simulink model "mount_2_rust"  (R2022b)
settings: Solver=FixedStepDiscrete  StartTime=0.0  StopTime=5  FixedStep=deltaT  RelTol=1e-3
InitFcn:
  | %
  | % Initialization callback function
  | %
  | 
  | try
  |    % fprintf('\n Simulink control model!\n');
  | 
  |    % Get Simulink model directory
  |    [filepath,name,ext] = fileparts(which(bdroot));
  | 
  |    if ~strcmp(filepath,pwd)
  |       fprintf('\n Changing current directory to \n %s \n',filepath);
  |       cd(filepath);
  |    end
  | 
  | catch
  |    warning('Running the InitFcn from puSimulate script');
  | end
values from neighbouring files (symbols this model uses):
  drv_delay = ceil(mount.delay/FEM_Ts)    [load_mount_data.m]
  FEM_Ts = deltaT    (= 0.000125)    [load_mount_data.m]
  Hdrive_d = c2d(o.Hdrive(1,1), FEM_Ts, 'tustin')    [load_mount_data.m]
  mnt_TF_Ts = FEM_Ts    (= 0.000125)    [load_mount_data.m]
  o = fun_confBase(oTest)    [load_mount_data.m]
undefined symbols (not defined in the file or in its folder): a, az, az_ff_en, b, c, DiscIntNeverNeededParam, el, gir, magnitude, mount
libraries: simulink x2, simulink_extras x2
(part 2 of 2)

== system mount_2_rust/Mount_Drv_PDR2021/ODC CT LUGRE Fr model/Friction ==
  Vel : Inport
  Enable : EnablePort
  Constant : Constant  Value=az.oFr.iIsActive
  Constant1 : Constant  Value=el.oFr.iIsActive
  Constant2 : Constant  Value=gir.oFr.iIsActive
  Demux1 : Demux  Outputs=3
  Friction Alt : Subsystem  mask{sigma0=el.oFr.sigm0, sigma1=el.oFr.sigm1, Tc=el.oFr.Tc, sigmav=el.oFr.sigmv, Ts=el.oFr.Ts, vs=el.oFr.vs, iIsSig01Active=el.oFr.iIsSig01Active}
      mask prompts: iIsSig01Active "0=inactive, 1=active"
  Friction Az : Subsystem  mask{sigma0=az.oFr.sigm0, sigma1=az.oFr.sigm1, Tc=az.oFr.Tc, sigmav=az.oFr.sigmv, Ts=az.oFr.Ts, vs=az.oFr.vs, iIsSig01Active=az.oFr.iIsSig01Active}
      mask prompts: iIsSig01Active "0=inactive, 1=active"
  Friction Gir : Subsystem  mask{sigma0=gir.oFr.sigm0, sigma1=gir.oFr.sigm1, Tc=gir.oFr.Tc, sigmav=gir.oFr.sigmv, Ts=gir.oFr.Ts, vs=gir.oFr.vs, iIsSig01Active=gir.oFr.iIsSig01Active}
      mask prompts: iIsSig01Active "0=inactive, 1=active"
  Mux2 : Mux  Inputs=3
  FrictionTo : Outport
  wires:
  Friction Gir/1(Tfr) -> Mux2/3
  Demux1/3 -> Friction Gir/1(v)
  Constant2/1 -> Friction Gir/Enable
  Constant/1 -> Friction Az/Enable
  Constant1/1 -> Friction Alt/Enable
  Mux2/1 -> FrictionTo/1
  Friction Az/1(Tfr) -> Mux2/1
  Demux1/1 -> Friction Az/1(v)
  Vel/1 -> Demux1/1
  Demux1/2 -> Friction Alt/1(v)
  Friction Alt/1(Tfr) -> Mux2/2

== system mount_2_rust/Mount_Drv_PDR2021/Parasitic torques model /AZ_Parasitic_Torque ==
  Drive_Pos : Inport
  Drive_Torque : Inport  Port=2
  Cogging : Lookup_n-D  NumberOfTableDimensions=1  LookupTableObject=F_ripple  BreakpointsForDimension1=ParasiticModelStruc.Pos  Table=ParasiticModelStruc.oCog.Amp  InternalRulePriority=Speed  RndMeth=Simplest
  Constant : Constant  Value=0.1869
  Divide : Product  Inputs=**
  EMF Distortion : Lookup_n-D  NumberOfTableDimensions=1  LookupTableObject=F_ripple  BreakpointsForDimension1=ParasiticModelStruc.Pos  Table=ParasiticModelStruc.oEmf.Amp  InternalRulePriority=Speed  RndMeth=Simplest
  Gain : Gain  Gain=1/ParasiticModelStruc.R
  Gain1 : Gain  Gain=1/250
  Gain2 : Gain  Gain=1/ParasiticModelStruc.N_Segm
  Mod : Math  Operator=rem  SignedPower=on
  Mod1 : Math  Operator=rem  SignedPower=on
  Radius : Gain  Gain=ParasiticModelStruc.R
  Sum1 : Sum
  Sum2 : Sum
  Parasitic_Torque : Outport  VectorParamsAs1DForOutWhenUnconnected=off
  wires:
  Sum1/1 -> Parasitic_Torque/1
  Drive_Pos/1 -> Radius/1  "Drive Position"
  Constant/1 -> Mod1/2, Sum2/2, Mod/2
  Gain2/1 -> Divide/1  "I_rms pro Segment"
  Mod/1 -> Sum2/1
  Sum2/1 -> Mod1/1
  EMF Distortion/1 -> Divide/2
  Gain/1 -> Gain1/1  "Force"
  Drive_Torque/1 -> Gain/1
  Radius/1 -> Mod/1  "driven  distance"
  Cogging/1 -> Sum1/2
  Mod1/1 -> Cogging/1, EMF Distortion/1
  Gain1/1 -> Gain2/1  "I_rms"
  Divide/1 -> Sum1/1

== system mount_2_rust/Mount_Drv_PDR2021/Parasitic torques model /EL_Parasitic_Torque ==
  Drive_Pos : Inport
  Drive_Torque : Inport  Port=2
  Cogging : Lookup_n-D  NumberOfTableDimensions=1  LookupTableObject=F_ripple  BreakpointsForDimension1=ParasiticModelStruc.Pos  Table=ParasiticModelStruc.oCog.Amp  InternalRulePriority=Speed  RndMeth=Simplest
  Constant : Constant  Value=0.1869
  Divide : Product  Inputs=**
  EMF Distortion : Lookup_n-D  NumberOfTableDimensions=1  LookupTableObject=F_ripple  BreakpointsForDimension1=ParasiticModelStruc.Pos  Table=ParasiticModelStruc.oEmf.Amp  InternalRulePriority=Speed  RndMeth=Simplest
  Gain : Gain  Gain=1/ParasiticModelStruc.R
  Gain1 : Gain  Gain=1/250
  Gain2 : Gain  Gain=1/ParasiticModelStruc.N_Segm
  Mod : Math  Operator=rem  SignedPower=on
  Mod1 : Math  Operator=rem  SignedPower=on
  Radius : Gain  Gain=ParasiticModelStruc.R
  Sum1 : Sum
  Sum2 : Sum
  Parasitic_Torque : Outport  VectorParamsAs1DForOutWhenUnconnected=off
  wires:
  Constant/1 -> Mod1/2, Sum2/2, Mod/2
  Divide/1 -> Sum1/1
  Mod1/1 -> Cogging/1, EMF Distortion/1
  Sum2/1 -> Mod1/1
  Radius/1 -> Mod/1  "driven  distance"
  Cogging/1 -> Sum1/2
  Mod/1 -> Sum2/1
  Gain/1 -> Gain1/1  "Force"
  Gain2/1 -> Divide/1  "I_rms pro Segment"
  Gain1/1 -> Gain2/1  "I_rms"
  Drive_Pos/1 -> Radius/1  "Drive Position"
  EMF Distortion/1 -> Divide/2
  Drive_Torque/1 -> Gain/1
  Sum1/1 -> Parasitic_Torque/1

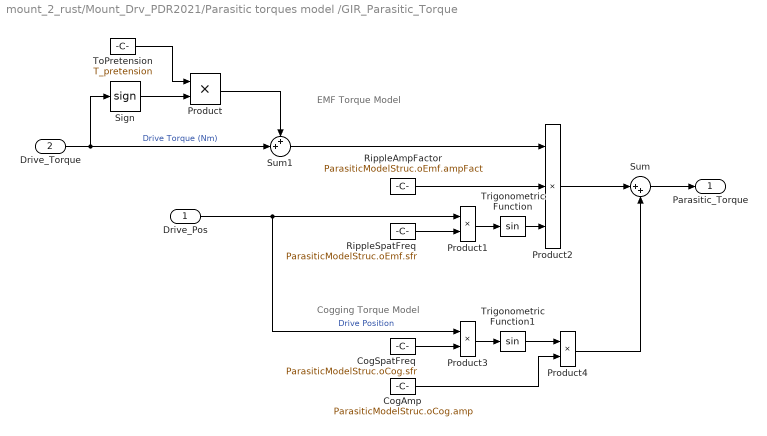
== system mount_2_rust/Mount_Drv_PDR2021/Parasitic torques model /GIR_Parasitic_Torque ==
  note: Cogging Torque Model
  note: EMF Torque Model
  Drive_Pos : Inport
  Drive_Torque : Inport  Port=2
  CogAmp : Constant  Value=ParasiticModelStruc.oCog.amp
  CogSpatFreq : Constant  Value=ParasiticModelStruc.oCog.sfr
  Product : Product
  Product1 : Product  RndMeth=Zero
  Product2 : Product  Inputs=3  RndMeth=Zero
  Product3 : Product  RndMeth=Zero
  Product4 : Product  RndMeth=Zero
  RippleAmpFactor : Constant  Value=ParasiticModelStruc.oEmf.ampFact
  RippleSpatFreq : Constant  Value=ParasiticModelStruc.oEmf.sfr
  Sign : Signum
  Sum : Sum  Inputs=|++
  Sum1 : Sum  Inputs=++|
  ToPretension : Constant  Value=T_pretension
  Trigonometric Function : Trigonometry
  Trigonometric Function1 : Trigonometry
  Parasitic_Torque : Outport  VectorParamsAs1DForOutWhenUnconnected=off
  wires:
  Product/1 -> Sum1/1
  ToPretension/1 -> Product/1
  Sign/1 -> Product/2
  Drive_Torque/1 -> Sum1/2, Sign/1  "Drive Torque (Nm)"
  Sum1/1 -> Product2/1
  Trigonometric Function/1 -> Product2/3
  Sum/1 -> Parasitic_Torque/1
  Product2/1 -> Sum/1
  Product4/1 -> Sum/2
  CogAmp/1 -> Product4/2
  Drive_Pos/1 -> Product1/1, Product3/1  "Drive Position"
  CogSpatFreq/1 -> Product3/2
  Trigonometric Function1/1 -> Product4/1
  Product3/1 -> Trigonometric Function1/1
  RippleSpatFreq/1 -> Product1/2
  Product1/1 -> Trigonometric Function/1
  RippleAmpFactor/1 -> Product2/2

== system mount_2_rust/Mount_Drv_PDR2021/Parasitic torques model /Subsystem ==
  Az Pos : Inport
  Az To : Inport  Port=2
  El Pos : Inport  Port=3
  El To : Inport  Port=4
  Gir Pos : Inport  Port=5
  Gir To : Inport  Port=6
  Constant2 : Constant
  Demux1 : Demux  Outputs=3
  Mux1 : Mux  Inputs=3
  Mux7 : Mux  Inputs=3
  Parasitic Torques : Subsystem
  Out1 : Outport  VectorParamsAs1DForOutWhenUnconnected=off
  Out2 : Outport  Port=2  VectorParamsAs1DForOutWhenUnconnected=off
  Out3 : Outport  Port=3  VectorParamsAs1DForOutWhenUnconnected=off
  wires:
  Gir To/1 -> Mux1/3
  El To/1 -> Mux1/2
  Az To/1 -> Mux1/1
  Parasitic Torques/1(ParasiticTo) -> Demux1/1
  El Pos/1 -> Mux7/2
  Constant2/1 -> Parasitic Torques/Enable
  Mux1/1 -> Parasitic Torques/1(MotTo)
  Mux7/1 -> Parasitic Torques/2(MotPos)
  Az Pos/1 -> Mux7/1
  Demux1/3 -> Out3/1
  Gir Pos/1 -> Mux7/3
  Demux1/2 -> Out2/1
  Demux1/1 -> Out1/1

== system mount_2_rust/Mount_Drv_PDR2021_Frless/Parasitic torques model /AZ_Parasitic_Torque ==
  Drive_Pos : Inport
  Drive_Torque : Inport  Port=2
  Cogging : Lookup_n-D  NumberOfTableDimensions=1  LookupTableObject=F_ripple  BreakpointsForDimension1=ParasiticModelStruc.Pos  Table=ParasiticModelStruc.oCog.Amp  InternalRulePriority=Speed  RndMeth=Simplest
  Constant : Constant  Value=0.1869
  Divide : Product  Inputs=**
  EMF Distortion : Lookup_n-D  NumberOfTableDimensions=1  LookupTableObject=F_ripple  BreakpointsForDimension1=ParasiticModelStruc.Pos  Table=ParasiticModelStruc.oEmf.Amp  InternalRulePriority=Speed  RndMeth=Simplest
  Gain : Gain  Gain=1/ParasiticModelStruc.R
  Gain1 : Gain  Gain=1/250
  Gain2 : Gain  Gain=1/ParasiticModelStruc.N_Segm
  Mod : Math  Operator=rem  SignedPower=on
  Mod1 : Math  Operator=rem  SignedPower=on
  Radius : Gain  Gain=ParasiticModelStruc.R
  Sum1 : Sum
  Sum2 : Sum
  Parasitic_Torque : Outport  VectorParamsAs1DForOutWhenUnconnected=off
  wires:
  Sum1/1 -> Parasitic_Torque/1
  Drive_Pos/1 -> Radius/1  "Drive Position"
  Constant/1 -> Mod1/2, Sum2/2, Mod/2
  Gain2/1 -> Divide/1  "I_rms pro Segment"
  Mod/1 -> Sum2/1
  Sum2/1 -> Mod1/1
  EMF Distortion/1 -> Divide/2
  Gain/1 -> Gain1/1  "Force"
  Drive_Torque/1 -> Gain/1
  Radius/1 -> Mod/1  "driven  distance"
  Cogging/1 -> Sum1/2
  Mod1/1 -> Cogging/1, EMF Distortion/1
  Gain1/1 -> Gain2/1  "I_rms"
  Divide/1 -> Sum1/1

== system mount_2_rust/Mount_Drv_PDR2021_Frless/Parasitic torques model /EL_Parasitic_Torque ==
  Drive_Pos : Inport
  Drive_Torque : Inport  Port=2
  Cogging : Lookup_n-D  NumberOfTableDimensions=1  LookupTableObject=F_ripple  BreakpointsForDimension1=ParasiticModelStruc.Pos  Table=ParasiticModelStruc.oCog.Amp  InternalRulePriority=Speed  RndMeth=Simplest
  Constant : Constant  Value=0.1869
  Divide : Product  Inputs=**
  EMF Distortion : Lookup_n-D  NumberOfTableDimensions=1  LookupTableObject=F_ripple  BreakpointsForDimension1=ParasiticModelStruc.Pos  Table=ParasiticModelStruc.oEmf.Amp  InternalRulePriority=Speed  RndMeth=Simplest
  Gain : Gain  Gain=1/ParasiticModelStruc.R
  Gain1 : Gain  Gain=1/250
  Gain2 : Gain  Gain=1/ParasiticModelStruc.N_Segm
  Mod : Math  Operator=rem  SignedPower=on
  Mod1 : Math  Operator=rem  SignedPower=on
  Radius : Gain  Gain=ParasiticModelStruc.R
  Sum1 : Sum
  Sum2 : Sum
  Parasitic_Torque : Outport  VectorParamsAs1DForOutWhenUnconnected=off
  wires:
  Constant/1 -> Mod1/2, Sum2/2, Mod/2
  Divide/1 -> Sum1/1
  Mod1/1 -> Cogging/1, EMF Distortion/1
  Sum2/1 -> Mod1/1
  Radius/1 -> Mod/1  "driven  distance"
  Cogging/1 -> Sum1/2
  Mod/1 -> Sum2/1
  Gain/1 -> Gain1/1  "Force"
  Gain2/1 -> Divide/1  "I_rms pro Segment"
  Gain1/1 -> Gain2/1  "I_rms"
  Drive_Pos/1 -> Radius/1  "Drive Position"
  EMF Distortion/1 -> Divide/2
  Drive_Torque/1 -> Gain/1
  Sum1/1 -> Parasitic_Torque/1

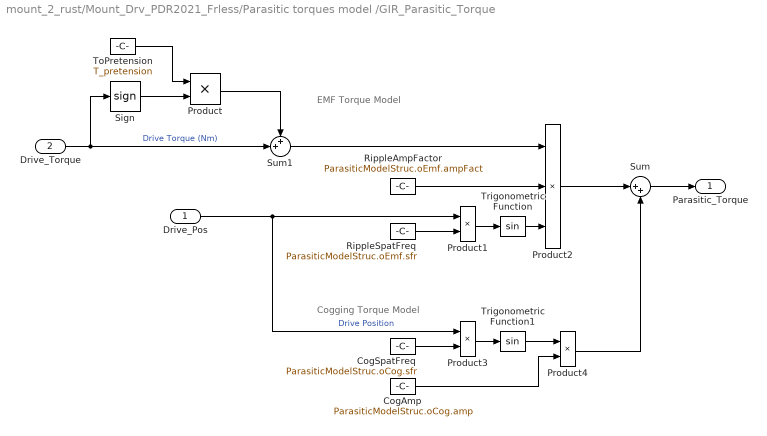
== system mount_2_rust/Mount_Drv_PDR2021_Frless/Parasitic torques model /GIR_Parasitic_Torque ==
  note: Cogging Torque Model
  note: EMF Torque Model
  Drive_Pos : Inport
  Drive_Torque : Inport  Port=2
  CogAmp : Constant  Value=ParasiticModelStruc.oCog.amp
  CogSpatFreq : Constant  Value=ParasiticModelStruc.oCog.sfr
  Product : Product
  Product1 : Product  RndMeth=Zero
  Product2 : Product  Inputs=3  RndMeth=Zero
  Product3 : Product  RndMeth=Zero
  Product4 : Product  RndMeth=Zero
  RippleAmpFactor : Constant  Value=ParasiticModelStruc.oEmf.ampFact
  RippleSpatFreq : Constant  Value=ParasiticModelStruc.oEmf.sfr
  Sign : Signum
  Sum : Sum  Inputs=|++
  Sum1 : Sum  Inputs=++|
  ToPretension : Constant  Value=T_pretension
  Trigonometric Function : Trigonometry
  Trigonometric Function1 : Trigonometry
  Parasitic_Torque : Outport  VectorParamsAs1DForOutWhenUnconnected=off
  wires:
  Product/1 -> Sum1/1
  ToPretension/1 -> Product/1
  Sign/1 -> Product/2
  Drive_Torque/1 -> Sum1/2, Sign/1  "Drive Torque (Nm)"
  Sum1/1 -> Product2/1
  Trigonometric Function/1 -> Product2/3
  Sum/1 -> Parasitic_Torque/1
  Product2/1 -> Sum/1
  Product4/1 -> Sum/2
  CogAmp/1 -> Product4/2
  Drive_Pos/1 -> Product1/1, Product3/1  "Drive Position"
  CogSpatFreq/1 -> Product3/2
  Trigonometric Function1/1 -> Product4/1
  Product3/1 -> Trigonometric Function1/1
  RippleSpatFreq/1 -> Product1/2
  Product1/1 -> Trigonometric Function/1
  RippleAmpFactor/1 -> Product2/2

== system mount_2_rust/Mount_Drv_PDR2021_Frless/Parasitic torques model /Subsystem ==
  Az Pos : Inport
  Az To : Inport  Port=2
  El Pos : Inport  Port=3
  El To : Inport  Port=4
  Gir Pos : Inport  Port=5
  Gir To : Inport  Port=6
  Constant2 : Constant
  Demux1 : Demux  Outputs=3
  Mux1 : Mux  Inputs=3
  Mux7 : Mux  Inputs=3
  Parasitic Torques : Subsystem
  Out1 : Outport  VectorParamsAs1DForOutWhenUnconnected=off
  Out2 : Outport  Port=2  VectorParamsAs1DForOutWhenUnconnected=off
  Out3 : Outport  Port=3  VectorParamsAs1DForOutWhenUnconnected=off
  wires:
  Gir To/1 -> Mux1/3
  El To/1 -> Mux1/2
  Az To/1 -> Mux1/1
  Parasitic Torques/1(ParasiticTo) -> Demux1/1
  El Pos/1 -> Mux7/2
  Constant2/1 -> Parasitic Torques/Enable
  Mux1/1 -> Parasitic Torques/1(MotTo)
  Mux7/1 -> Parasitic Torques/2(MotPos)
  Az Pos/1 -> Mux7/1
  Demux1/3 -> Out3/1
  Gir Pos/1 -> Mux7/3
  Demux1/2 -> Out2/1
  Demux1/1 -> Out1/1

== system mount_2_rust/Mount_Drv_FDR2023/DRV Friction/AZ DT Lugre Fr mode/g(v) ==
  v : Inport
  Enable : EnablePort
  Constant : Constant  Value=0
  Sum : Sum  Inputs=|++
  gc : Constant  Value=Tc/sigma0
  gs : Subsystem
  g : Outport
  wires:
  Constant/1 -> gs/Enable
  gc/1 -> Sum/2
  gs/1(gs(v)) -> Sum/1
  v/1 -> gs/1(v)
  Sum/1 -> g/1

== system mount_2_rust/Mount_Drv_FDR2023/DRV Friction/AZ DT Lugre Fr mode/v2z ==
  v : Inport
  g(v) : Inport  Port=2
  z : Inport  Port=3
  Enable : EnablePort
  Abs : Abs  SaturateOnIntegerOverflow=off
  Divide : Product  Inputs=*/*
  Sum : Sum  Inputs=|+-
  dz : Outport
  wires:
  z/1 -> Divide/3
  g(v)/1 -> Divide/2
  Sum/1 -> dz/1
  v/1 -> Abs/1, Sum/1
  Divide/1 -> Sum/2
  Abs/1 -> Divide/1

== system mount_2_rust/Mount_Drv_FDR2023/DRV Friction/EL DT Lugre Fr model/g(v) ==
  v : Inport
  Enable : EnablePort
  Constant : Constant  Value=0
  Sum : Sum  Inputs=|++
  gc : Constant  Value=Tc/sigma0
  gs : Subsystem
  g : Outport
  wires:
  Constant/1 -> gs/Enable
  gc/1 -> Sum/2
  gs/1(gs(v)) -> Sum/1
  v/1 -> gs/1(v)
  Sum/1 -> g/1

== system mount_2_rust/Mount_Drv_FDR2023/DRV Friction/EL DT Lugre Fr model/v2z ==
  v : Inport
  g(v) : Inport  Port=2
  z : Inport  Port=3
  Enable : EnablePort
  Abs : Abs  SaturateOnIntegerOverflow=off
  Divide : Product  Inputs=*/*
  Sum : Sum  Inputs=|+-
  dz : Outport
  wires:
  z/1 -> Divide/3
  g(v)/1 -> Divide/2
  Sum/1 -> dz/1
  v/1 -> Abs/1, Sum/1
  Divide/1 -> Sum/2
  Abs/1 -> Divide/1

== system mount_2_rust/Mount_Drv_FDR2023/DRV Friction/EL DT Lugre Fr model_/g(v) ==
  v : Inport
  Enable : EnablePort
  Constant : Constant  Value=0
  Sum : Sum  Inputs=|++
  gc : Constant  Value=frParStruct.Tc/frParStruct.sigm0
  gs : Subsystem
  g : Outport  VectorParamsAs1DForOutWhenUnconnected=off
  wires:
  Constant/1 -> gs/Enable
  gc/1 -> Sum/2
  gs/1(gs(v)) -> Sum/1
  v/1 -> gs/1(v)
  Sum/1 -> g/1

== system mount_2_rust/Mount_Drv_FDR2023/DRV Friction/EL DT Lugre Fr model_/v2z ==
  v : Inport
  g(v) : Inport  Port=2
  z : Inport  Port=3
  Enable : EnablePort
  Abs : Abs  SaturateOnIntegerOverflow=off
  Divide : Product  Inputs=*/*
  Sum : Sum  Inputs=|+-
  dz : Outport  VectorParamsAs1DForOutWhenUnconnected=off
  wires:
  z/1 -> Divide/3
  g(v)/1 -> Divide/2
  Sum/1 -> dz/1
  v/1 -> Abs/1, Sum/1
  Divide/1 -> Sum/2
  Abs/1 -> Divide/1

== system mount_2_rust/Mount_Drv_FDR2023/DRV Friction/GIR DT Lugre Fr model/g(v) ==
  v : Inport
  Constant : Constant  Value=0
  Sum : Sum  Inputs=|++
  gc : Constant  Value=Tc/sigma0
  gs : Subsystem
  g : Outport
  wires:
  Constant/1 -> gs/Enable
  gc/1 -> Sum/2
  gs/1(gs(v)) -> Sum/1
  v/1 -> gs/1(v)
  Sum/1 -> g/1

== system mount_2_rust/Mount_Drv_FDR2023/DRV Friction/GIR DT Lugre Fr model/v2z ==
  v : Inport
  g(v) : Inport  Port=2
  z : Inport  Port=3
  Abs : Abs  SaturateOnIntegerOverflow=off
  Divide : Product  Inputs=*/*
  Sum : Sum  Inputs=|+-
  dz : Outport
  wires:
  z/1 -> Divide/3
  g(v)/1 -> Divide/2
  Sum/1 -> dz/1
  v/1 -> Abs/1, Sum/1
  Divide/1 -> Sum/2
  Abs/1 -> Divide/1

== system mount_2_rust/Mount_Drv_FDR2023/DRV Friction/GIR DT Lugre Fr model_/g(v) ==
  v : Inport
  Constant : Constant  Value=0
  Sum : Sum  Inputs=|++
  gc : Constant  Value=frParStruct.Tc/frParStruct.sigm0
  gs : Subsystem
  g : Outport  VectorParamsAs1DForOutWhenUnconnected=off
  wires:
  Constant/1 -> gs/Enable
  gc/1 -> Sum/2
  gs/1(gs(v)) -> Sum/1
  v/1 -> gs/1(v)
  Sum/1 -> g/1

== system mount_2_rust/Mount_Drv_FDR2023/DRV Friction/GIR DT Lugre Fr model_/v2z ==
  note: $\text{Let}\\ |v| = v \sign(v) \\ \text{Sign function approximation:}\\ S_0(v) = \frac{2}{\pi}\atan(k_v v) \\ \text{Then, one approximates the original LuGre model equation}\\ \dot{z} = v - \frac{|v|}{g(v)}z \\ \text{with} \\ \dot{z} = vS_0^2(v) - \frac{vS_0(v)}{g(v)}z .$
  note: Original implementation
  v : Inport
  g(v) : Inport  Port=2
  z : Inport  Port=3
  2/pi : Gain  Gain=2/pi
  Abs1 : Abs  SaturateOnIntegerOverflow=off
  Divide : Product  Inputs=*/*
  Divide1 : Product  Inputs=*/*
  Divide2 : Product  Inputs=**
  Divide3 : Product  Inputs=**
  Math Function : Math  Operator=square  SignedPower=on
  Smoothed-Discontinuous Lugre Model Switch : ManualSwitch
  Sum : Sum  Inputs=|+-
  Sum1 : Sum  Inputs=|+-
  Trigonometric Function : Trigonometry  Operator=atan
  kv : Gain  Gain=1e6%1e-6
  dz : Outport  VectorParamsAs1DForOutWhenUnconnected=off
  wires:
  Smoothed-Discontinuous Lugre Model Switch/1 -> dz/1
  Sum/1 -> Smoothed-Discontinuous Lugre Model Switch/1  "Smoothed Lugre"
  Divide2/1 -> Sum/1
  Divide3/1 -> Divide/1  "S_2"
  Math Function/1 -> Divide2/2  "S_1"
  2/pi/1 -> Math Function/1, Divide3/1  "S_0"
  kv/1 -> Trigonometric Function/1
  Trigonometric Function/1 -> 2/pi/1
  v/1 -> Divide2/1, kv/1, Divide3/2, Sum1/1, Abs1/1
  z/1 -> Divide/3, Divide1/3
  Sum1/1 -> Smoothed-Discontinuous Lugre Model Switch/2  "Discontinuous"
  Abs1/1 -> Divide1/1
  g(v)/1 -> Divide/2, Divide1/2
  Divide1/1 -> Sum1/2
  Divide/1 -> Sum/2

== system mount_2_rust/Mount_Drv_FDR2023/Parasitic torque model/Parasitic AZ/For Each Subsystem ==
  In1 : Inport  Partition=on  PartitionDimension=1  PartitionWidth=1  PartitionOffset=0
  EMF Spatial Pattern (N/A) : Sin  TimeSource=Use external signal  Amplitude=oParasitic.oEmf.SpAmp_NPerA  Frequency=oParasitic.oEmf.SpFreq_mmInv*2*pi  Phase=oParasitic.oEmf.SpPhase_rad  SampleTime=0
  For Each : ForEach  DisableCoverage=on
  Sum of Elements2 : Sum  Inputs=+
  Out1 : Outport  ConcatenationDimension=1
  wires:
  Sum of Elements2/1 -> Out1/1
  In1/1 -> EMF Spatial Pattern (N/A)/1
  EMF Spatial Pattern (N/A)/1 -> Sum of Elements2/1

== system mount_2_rust/Mount_Drv_FDR2023/Parasitic torque model/Parasitic AZ/For Each Subsystem1 ==
  In1 : Inport  Partition=on  PartitionDimension=1  PartitionWidth=1  PartitionOffset=0
  Cogging Spatial Pattern (N) : Sin  TimeSource=Use external signal  Amplitude=oParasitic.oCog.SpAmp_N  Frequency=oParasitic.oCog.SpFreq_mmInv*2*pi  Phase=oParasitic.oCog.SpPhase_rad  SampleTime=0
  For Each : ForEach  DisableCoverage=on
  Sum of Elements2 : Sum  Inputs=+
  Out1 : Outport  ConcatenationDimension=1
  wires:
  Sum of Elements2/1 -> Out1/1
  In1/1 -> Cogging Spatial Pattern (N)/1
  Cogging Spatial Pattern (N)/1 -> Sum of Elements2/1

== system mount_2_rust/Mount_Drv_FDR2023/Parasitic torque model/Parasitic EL/For Each Subsystem ==
  In1 : Inport  Partition=on  PartitionDimension=1  PartitionWidth=1  PartitionOffset=0
  EMF Spatial Pattern (N/A) : Sin  TimeSource=Use external signal  Amplitude=oParasitic.oEmf.SpAmp_NPerA  Frequency=oParasitic.oEmf.SpFreq_mmInv*2*pi  Phase=oParasitic.oEmf.SpPhase_rad  SampleTime=0
  For Each : ForEach  DisableCoverage=on
  Sum of Elements2 : Sum  Inputs=+
  Out1 : Outport  ConcatenationDimension=1
  wires:
  Sum of Elements2/1 -> Out1/1
  In1/1 -> EMF Spatial Pattern (N/A)/1
  EMF Spatial Pattern (N/A)/1 -> Sum of Elements2/1

== system mount_2_rust/Mount_Drv_FDR2023/Parasitic torque model/Parasitic EL/For Each Subsystem1 ==
  In1 : Inport  Partition=on  PartitionDimension=1  PartitionWidth=1  PartitionOffset=0
  Cogging Spatial Pattern (N) : Sin  TimeSource=Use external signal  Amplitude=oParasitic.oCog.SpAmp_N  Frequency=oParasitic.oCog.SpFreq_mmInv*2*pi  Phase=oParasitic.oCog.SpPhase_rad  SampleTime=0
  For Each : ForEach  DisableCoverage=on
  Sum of Elements2 : Sum  Inputs=+
  Out1 : Outport  ConcatenationDimension=1
  wires:
  Sum of Elements2/1 -> Out1/1
  In1/1 -> Cogging Spatial Pattern (N)/1
  Cogging Spatial Pattern (N)/1 -> Sum of Elements2/1

== system mount_2_rust/Mount_Drv_FDR2023/Parasitic torque model/Parasitic GIR/For Each Subsystem ==
  In1 : Inport  Partition=on  PartitionDimension=1  PartitionWidth=1  PartitionOffset=0
  (N/A) : Sin  TimeSource=Use external signal  Amplitude=oParasitic.oEmf.SpAmp_NmPerA  Frequency=oParasitic.oEmf.SpFreq_degInv*2*pi  Phase=oParasitic.oEmf.SpPhase_rad  SampleTime=0
  For Each : ForEach  DisableCoverage=on
  Sum of Elements2 : Sum  Inputs=+
  Out1 : Outport  ConcatenationDimension=1
  wires:
  Sum of Elements2/1 -> Out1/1
  In1/1 -> (N/A)/1
  (N/A)/1 -> Sum of Elements2/1

== system mount_2_rust/Mount_Drv_FDR2023/Parasitic torque model/Parasitic GIR/For Each Subsystem1 ==
  In1 : Inport  Partition=on  PartitionDimension=1  PartitionWidth=1  PartitionOffset=0
  Cogging Spatial Pattern (N) : Sin  TimeSource=Use external signal  Amplitude=oParasitic.oCog.SpAmp_Nm  Frequency=oParasitic.oCog.SpFreq_degInv*2*pi  Phase=oParasitic.oCog.SpPhase_rad  SampleTime=0
  For Each : ForEach  DisableCoverage=on
  Sum of Elements2 : Sum  Inputs=+
  Out1 : Outport  ConcatenationDimension=1
  wires:
  Sum of Elements2/1 -> Out1/1
  In1/1 -> Cogging Spatial Pattern (N)/1
  Cogging Spatial Pattern (N)/1 -> Sum of Elements2/1

== system mount_2_rust/Mount_Drv_PDR2021/AZ DT Lugre Fr model/g(v)/gs ==
  v : Inport
  Enable : EnablePort
  Divide : Product  Inputs=**
  Gain : Gain  Gain=1/frParStruct.vs
  Math Function : Math  SignedPower=on
  Math Function1 : Math  Operator=magnitude^2  SignedPower=on
  Sum : Sum  Inputs=|++
  Unary Minus : UnaryMinus
  gc : Constant  Value=frParStruct.Tc/frParStruct.sigm0
  gs : Constant  Value=(frParStruct.Ts-frParStruct.Tc)/frParStruct.sigm0
  gs(v) : Outport  VectorParamsAs1DForOutWhenUnconnected=off
  wires:
  Sum/1 -> gs(v)/1
  Divide/1 -> Sum/1
  gc/1 -> Sum/2
  v/1 -> Gain/1
  Gain/1 -> Math Function1/1
  Unary Minus/1 -> Math Function/1
  Math Function1/1 -> Unary Minus/1
  gs/1 -> Divide/2
  Math Function/1 -> Divide/1

== system mount_2_rust/Mount_Drv_PDR2021/EL DT Lugre Fr model/g(v)/gs ==
  v : Inport
  Enable : EnablePort
  Divide : Product  Inputs=**
  Gain : Gain  Gain=1/frParStruct.vs
  Math Function : Math  SignedPower=on
  Math Function1 : Math  Operator=magnitude^2  SignedPower=on
  Unary Minus : UnaryMinus
  gs : Constant  Value=(frParStruct.Ts-frParStruct.Tc)/frParStruct.sigm0
  gs(v) : Outport  VectorParamsAs1DForOutWhenUnconnected=off
  wires:
  Divide/1 -> gs(v)/1
  v/1 -> Gain/1
  Gain/1 -> Math Function1/1
  Unary Minus/1 -> Math Function/1
  Math Function1/1 -> Unary Minus/1
  gs/1 -> Divide/2
  Math Function/1 -> Divide/1

== system mount_2_rust/Mount_Drv_PDR2021/GIR DT Lugre Fr model/g(v)/gs ==
  v : Inport
  Enable : EnablePort
  Divide : Product  Inputs=**
  Gain : Gain  Gain=1/frParStruct.vs
  Math Function : Math  SignedPower=on
  Math Function1 : Math  Operator=magnitude^2  SignedPower=on
  Unary Minus : UnaryMinus
  gs : Constant  Value=(frParStruct.Ts-frParStruct.Tc)/frParStruct.sigm0
  gs(v) : Outport  VectorParamsAs1DForOutWhenUnconnected=off
  wires:
  Divide/1 -> gs(v)/1
  v/1 -> Gain/1
  Gain/1 -> Math Function1/1
  Unary Minus/1 -> Math Function/1
  Math Function1/1 -> Unary Minus/1
  gs/1 -> Divide/2
  Math Function/1 -> Divide/1

== system mount_2_rust/Mount_Drv_PDR2021/ODC CT LUGRE Fr model/Friction/Friction Alt ==
  v : Inport
  Enable : EnablePort
  Constant : Constant  Value=iIsSig01Active
  Integrator2 : Integrator
  Sum : Sum  Inputs=+++
  g(v) : Subsystem
  sigma_0 : Gain  Gain=sigma0
  sigma_1 : Gain  Gain=sigma1
  sigma_v : Gain  Gain=sigmav
  v2z : Subsystem
  Tfr : Outport
  wires:
  Constant/1 -> g(v)/Enable, v2z/Enable
  v/1 -> sigma_v/1, v2z/1(v), g(v)/1(v)
  sigma_v/1 -> Sum/3
  sigma_1/1 -> Sum/1
  Sum/1 -> Tfr/1
  sigma_0/1 -> Sum/2
  g(v)/1(g) -> v2z/2(g(v))
  Integrator2/1 -> v2z/3(z), sigma_0/1
  v2z/1(dz) -> sigma_1/1, Integrator2/1

== system mount_2_rust/Mount_Drv_PDR2021/ODC CT LUGRE Fr model/Friction/Friction Az ==
  v : Inport
  Enable : EnablePort
  Constant : Constant  Value=iIsSig01Active
  Integrator2 : Integrator
  Sum : Sum  Inputs=+++
  g(v) : Subsystem
  sigma_0 : Gain  Gain=sigma0
  sigma_1 : Gain  Gain=sigma1
  sigma_v : Gain  Gain=sigmav
  v2z : Subsystem
  Tfr : Outport
  wires:
  Constant/1 -> v2z/Enable, g(v)/Enable
  v/1 -> sigma_v/1, v2z/1(v), g(v)/1(v)
  sigma_v/1 -> Sum/3
  sigma_1/1 -> Sum/1
  Sum/1 -> Tfr/1
  sigma_0/1 -> Sum/2
  g(v)/1(g) -> v2z/2(g(v))
  Integrator2/1 -> v2z/3(z), sigma_0/1
  v2z/1(dz) -> sigma_1/1, Integrator2/1

== system mount_2_rust/Mount_Drv_PDR2021/ODC CT LUGRE Fr model/Friction/Friction Gir ==
  v : Inport
  Enable : EnablePort
  Integrator2 : Integrator
  Sum : Sum  Inputs=+++
  g(v) : Subsystem
  iIsSig01Active : Gain  Gain=iIsSig01Active
  sigma_0 : Gain  Gain=sigma0
  sigma_1 : Gain  Gain=sigma1
  sigma_v : Gain  Gain=sigmav
  v2z : Subsystem
  Tfr : Outport
  wires:
  iIsSig01Active/1 -> v2z/1(v), g(v)/1(v)
  sigma_v/1 -> Sum/3
  sigma_1/1 -> Sum/1
  Sum/1 -> Tfr/1
  sigma_0/1 -> Sum/2
  g(v)/1(g) -> v2z/2(g(v))
  Integrator2/1 -> v2z/3(z), sigma_0/1
  v/1 -> iIsSig01Active/1, sigma_v/1
  v2z/1(dz) -> sigma_1/1, Integrator2/1

== system mount_2_rust/Mount_Drv_PDR2021/Parasitic torques model /Subsystem/Parasitic Torques ==
  MotTo : Inport
  MotPos : Inport  Port=2
  Enable : EnablePort
  Demux1 : Demux  Outputs=2
  Demux2 : Demux  Outputs=2
  Demux3 : Demux  Outputs=2
  Mux2 : Mux  Inputs=2
  Mux3 : Mux  Inputs=3
  Parasitic AZ : Subsystem  mask{Pos=az.oParasitic.Pos, Amp_Cog=az.oParasitic.oCog.Amp, Amp_EMF=az.oParasitic.oEmf.Amp, R=az.oParasitic.R, N_Segm=az.oParasitic.N_Segm}
  Parasitic EL : Subsystem  mask{Pos=el.oParasitic.Pos, Amp_Cog=el.oParasitic.oCog.Amp, Amp_EMF=el.oParasitic.oEmf.Amp, R=el.oParasitic.R, N_Segm=el.oParasitic.N_Segm}
  Parasitic GIR : Subsystem  mask{cog_sfr=gir.oParasitic.oCog.sfr, cog_amp=gir.oParasitic.oCog.amp, emf_sfr=gir.oParasitic.oEmf.sfr, emf_ampFact=gir.oParasitic.oEmf.ampFact, T_pretension=gir.T_pretension}
  Sel : Selector  InputPortWidth=6  IndexOptions=Index vector (dialog)  Indices=[1 4]  OutputSizes=1
  Sel1 : Selector  InputPortWidth=6  IndexOptions=Index vector (dialog)  Indices=[2 5]  OutputSizes=1
  Sel2 : Selector  InputPortWidth=6  IndexOptions=Index vector (dialog)  Indices=[3 6]  OutputSizes=1
  ParasiticTo : Outport
  wires:
  Parasitic GIR/1(To) -> Mux3/3
  Demux1/1 -> Parasitic EL/1(MotTo)
  Demux3/1 -> Parasitic AZ/1(MotTo)
  Sel2/1 -> Demux2/1
  Demux2/2 -> Parasitic GIR/2(MotPos)
  Demux2/1 -> Parasitic GIR/1(MotTo)
  Parasitic EL/1(To) -> Mux3/2
  Demux1/2 -> Parasitic EL/2(MotPos)
  Sel1/1 -> Demux1/1
  Parasitic AZ/1(To) -> Mux3/1
  Demux3/2 -> Parasitic AZ/2(MotPos)
  Sel/1 -> Demux3/1
  MotPos/1 -> Mux2/2
  MotTo/1 -> Mux2/1
  Mux2/1 -> Sel1/1, Sel2/1, Sel/1
  Mux3/1 -> ParasiticTo/1

== system mount_2_rust/Mount_Drv_PDR2021_Frless/Parasitic torques model /Subsystem/Parasitic Torques ==
  MotTo : Inport
  MotPos : Inport  Port=2
  Enable : EnablePort
  Demux1 : Demux  Outputs=2
  Demux2 : Demux  Outputs=2
  Demux3 : Demux  Outputs=2
  Mux2 : Mux  Inputs=2
  Mux3 : Mux  Inputs=3
  Parasitic AZ : Subsystem  mask{Pos=az.oParasitic.Pos, Amp_Cog=az.oParasitic.oCog.Amp, Amp_EMF=az.oParasitic.oEmf.Amp, R=az.oParasitic.R, N_Segm=az.oParasitic.N_Segm}
  Parasitic EL : Subsystem  mask{Pos=el.oParasitic.Pos, Amp_Cog=el.oParasitic.oCog.Amp, Amp_EMF=el.oParasitic.oEmf.Amp, R=el.oParasitic.R, N_Segm=el.oParasitic.N_Segm}
  Parasitic GIR : Subsystem  mask{cog_sfr=gir.oParasitic.oCog.sfr, cog_amp=gir.oParasitic.oCog.amp, emf_sfr=gir.oParasitic.oEmf.sfr, emf_ampFact=gir.oParasitic.oEmf.ampFact, T_pretension=gir.T_pretension}
  Sel : Selector  InputPortWidth=6  IndexOptions=Index vector (dialog)  Indices=[1 4]  OutputSizes=1
  Sel1 : Selector  InputPortWidth=6  IndexOptions=Index vector (dialog)  Indices=[2 5]  OutputSizes=1
  Sel2 : Selector  InputPortWidth=6  IndexOptions=Index vector (dialog)  Indices=[3 6]  OutputSizes=1
  ParasiticTo : Outport
  wires:
  Parasitic GIR/1(To) -> Mux3/3
  Demux1/1 -> Parasitic EL/1(MotTo)
  Demux3/1 -> Parasitic AZ/1(MotTo)
  Sel2/1 -> Demux2/1
  Demux2/2 -> Parasitic GIR/2(MotPos)
  Demux2/1 -> Parasitic GIR/1(MotTo)
  Parasitic EL/1(To) -> Mux3/2
  Demux1/2 -> Parasitic EL/2(MotPos)
  Sel1/1 -> Demux1/1
  Parasitic AZ/1(To) -> Mux3/1
  Demux3/2 -> Parasitic AZ/2(MotPos)
  Sel/1 -> Demux3/1
  MotPos/1 -> Mux2/2
  MotTo/1 -> Mux2/1
  Mux2/1 -> Sel1/1, Sel2/1, Sel/1
  Mux3/1 -> ParasiticTo/1

== system mount_2_rust/Mount_Drv_FDR2023/DRV Friction/AZ DT Lugre Fr mode/g(v)/gs ==
  v : Inport
  Enable : EnablePort
  Divide : Product  Inputs=**
  Gain : Gain  Gain=1/vs
  Math Function : Math  SignedPower=on
  Math Function1 : Math  Operator=magnitude^2  SignedPower=on
  Unary Minus : UnaryMinus
  gs : Constant  Value=(Ts-Tc)/sigma0
  gs(v) : Outport
  wires:
  Divide/1 -> gs(v)/1
  v/1 -> Gain/1
  Gain/1 -> Math Function1/1
  Unary Minus/1 -> Math Function/1
  Math Function1/1 -> Unary Minus/1
  gs/1 -> Divide/2
  Math Function/1 -> Divide/1

== system mount_2_rust/Mount_Drv_FDR2023/DRV Friction/EL DT Lugre Fr model/g(v)/gs ==
  v : Inport
  Enable : EnablePort
  Divide : Product  Inputs=**
  Gain : Gain  Gain=1/vs
  Math Function : Math  SignedPower=on
  Math Function1 : Math  Operator=magnitude^2  SignedPower=on
  Unary Minus : UnaryMinus
  gs : Constant  Value=(Ts-Tc)/sigma0
  gs(v) : Outport
  wires:
  Divide/1 -> gs(v)/1
  v/1 -> Gain/1
  Gain/1 -> Math Function1/1
  Unary Minus/1 -> Math Function/1
  Math Function1/1 -> Unary Minus/1
  gs/1 -> Divide/2
  Math Function/1 -> Divide/1

== system mount_2_rust/Mount_Drv_FDR2023/DRV Friction/EL DT Lugre Fr model_/g(v)/gs ==
  v : Inport
  Enable : EnablePort
  Divide : Product  Inputs=**
  Gain : Gain  Gain=1/frParStruct.vs
  Math Function : Math  SignedPower=on
  Math Function1 : Math  Operator=magnitude^2  SignedPower=on
  Unary Minus : UnaryMinus
  gs : Constant  Value=(frParStruct.Ts-frParStruct.Tc)/frParStruct.sigm0
  gs(v) : Outport  VectorParamsAs1DForOutWhenUnconnected=off
  wires:
  Divide/1 -> gs(v)/1
  v/1 -> Gain/1
  Gain/1 -> Math Function1/1
  Unary Minus/1 -> Math Function/1
  Math Function1/1 -> Unary Minus/1
  gs/1 -> Divide/2
  Math Function/1 -> Divide/1

== system mount_2_rust/Mount_Drv_FDR2023/DRV Friction/GIR DT Lugre Fr model/g(v)/gs ==
  v : Inport
  Enable : EnablePort
  Divide : Product  Inputs=**
  Gain : Gain  Gain=1/vs
  Math Function : Math  SignedPower=on
  Math Function1 : Math  Operator=magnitude^2  SignedPower=on
  Unary Minus : UnaryMinus
  gs : Constant  Value=(Ts-Tc)/sigma0
  gs(v) : Outport
  wires:
  Divide/1 -> gs(v)/1
  v/1 -> Gain/1
  Gain/1 -> Math Function1/1
  Unary Minus/1 -> Math Function/1
  Math Function1/1 -> Unary Minus/1
  gs/1 -> Divide/2
  Math Function/1 -> Divide/1

== system mount_2_rust/Mount_Drv_FDR2023/DRV Friction/GIR DT Lugre Fr model_/g(v)/gs ==
  v : Inport
  Enable : EnablePort
  Divide : Product  Inputs=**
  Gain : Gain  Gain=1/frParStruct.vs
  Math Function : Math  SignedPower=on
  Math Function1 : Math  Operator=magnitude^2  SignedPower=on
  Unary Minus : UnaryMinus
  gs : Constant  Value=(frParStruct.Ts-frParStruct.Tc)/frParStruct.sigm0
  gs(v) : Outport  VectorParamsAs1DForOutWhenUnconnected=off
  wires:
  Divide/1 -> gs(v)/1
  v/1 -> Gain/1
  Gain/1 -> Math Function1/1
  Unary Minus/1 -> Math Function/1
  Math Function1/1 -> Unary Minus/1
  gs/1 -> Divide/2
  Math Function/1 -> Divide/1

== system mount_2_rust/Mount_Drv_PDR2021/ODC CT LUGRE Fr model/Friction/Friction Alt/g(v) ==
  v : Inport
  Enable : EnablePort
  Constant : Constant  Value=0
  Sum : Sum  Inputs=|++
  gc : Constant  Value=Tc/sigma0
  gs : Subsystem
  g : Outport
  wires:
  Constant/1 -> gs/Enable
  gc/1 -> Sum/2
  gs/1(gs(v)) -> Sum/1
  v/1 -> gs/1(v)
  Sum/1 -> g/1

== system mount_2_rust/Mount_Drv_PDR2021/ODC CT LUGRE Fr model/Friction/Friction Alt/v2z ==
  v : Inport
  g(v) : Inport  Port=2
  z : Inport  Port=3
  Enable : EnablePort
  Abs : Abs  SaturateOnIntegerOverflow=off
  Divide : Product  Inputs=*/*
  Sum : Sum  Inputs=|+-
  dz : Outport
  wires:
  z/1 -> Divide/3
  g(v)/1 -> Divide/2
  Sum/1 -> dz/1
  v/1 -> Abs/1, Sum/1
  Divide/1 -> Sum/2
  Abs/1 -> Divide/1

== system mount_2_rust/Mount_Drv_PDR2021/ODC CT LUGRE Fr model/Friction/Friction Az/g(v) ==
  v : Inport
  Enable : EnablePort
  Constant : Constant  Value=0
  Sum : Sum  Inputs=|++
  gc : Constant  Value=Tc/sigma0
  gs : Subsystem
  g : Outport
  wires:
  Constant/1 -> gs/Enable
  gc/1 -> Sum/2
  gs/1(gs(v)) -> Sum/1
  v/1 -> gs/1(v)
  Sum/1 -> g/1

== system mount_2_rust/Mount_Drv_PDR2021/ODC CT LUGRE Fr model/Friction/Friction Az/v2z ==
  v : Inport
  g(v) : Inport  Port=2
  z : Inport  Port=3
  Enable : EnablePort
  Abs : Abs  SaturateOnIntegerOverflow=off
  Divide : Product  Inputs=*/*
  Sum : Sum  Inputs=|+-
  dz : Outport
  wires:
  z/1 -> Divide/3
  g(v)/1 -> Divide/2
  Sum/1 -> dz/1
  v/1 -> Abs/1, Sum/1
  Divide/1 -> Sum/2
  Abs/1 -> Divide/1

== system mount_2_rust/Mount_Drv_PDR2021/ODC CT LUGRE Fr model/Friction/Friction Gir/g(v) ==
  v : Inport
  Constant : Constant  Value=0
  Sum : Sum  Inputs=|++
  gc : Constant  Value=Tc/sigma0
  gs : Subsystem
  g : Outport
  wires:
  Constant/1 -> gs/Enable
  gc/1 -> Sum/2
  gs/1(gs(v)) -> Sum/1
  v/1 -> gs/1(v)
  Sum/1 -> g/1

== system mount_2_rust/Mount_Drv_PDR2021/ODC CT LUGRE Fr model/Friction/Friction Gir/v2z ==
  v : Inport
  g(v) : Inport  Port=2
  z : Inport  Port=3
  Abs : Abs  SaturateOnIntegerOverflow=off
  Divide : Product  Inputs=*/*
  Sum : Sum  Inputs=|+-
  dz : Outport
  wires:
  z/1 -> Divide/3
  g(v)/1 -> Divide/2
  Sum/1 -> dz/1
  v/1 -> Abs/1, Sum/1
  Divide/1 -> Sum/2
  Abs/1 -> Divide/1

== system mount_2_rust/Mount_Drv_PDR2021/Parasitic torques model /Subsystem/Parasitic Torques/Parasitic AZ ==
  MotTo : Inport
  MotPos : Inport  Port=2
  Cogging : Lookup_n-D  NumberOfTableDimensions=1  LookupTableObject=F_ripple  BreakpointsForDimension1=Pos  Table=Amp_Cog  InternalRulePriority=Speed  RndMeth=Simplest
  Constant : Constant  Value=0.1869
  Divide : Product  Inputs=**
  EMF Distortion : Lookup_n-D  NumberOfTableDimensions=1  LookupTableObject=F_ripple  BreakpointsForDimension1=Pos  Table=Amp_EMF  InternalRulePriority=Speed  RndMeth=Simplest
  Gain : Gain  Gain=1/R
  Gain1 : Gain  Gain=1/250
  Gain2 : Gain  Gain=1/N_Segm
  Mod : Math  Operator=rem  SignedPower=on
  Mod1 : Math  Operator=rem  SignedPower=on
  Radius : Gain  Gain=R
  Sum : Sum  Inputs=|++
  Sum1 : Sum  Inputs=|++
  To : Outport
  wires:
  Mod1/1 -> Cogging/1, EMF Distortion/1
  Sum1/1 -> Mod1/1
  Mod/1 -> Sum1/1
  Gain1/1 -> Gain2/1  "I_rms"
  Gain2/1 -> Divide/1  "I_rms pro Segment"
  Divide/1 -> Sum/1
  EMF Distortion/1 -> Divide/2
  Gain/1 -> Gain1/1  "Force"
  MotTo/1 -> Gain/1
  Cogging/1 -> Sum/2
  Sum/1 -> To/1
  MotPos/1 -> Radius/1
  Constant/1 -> Mod/2, Sum1/2, Mod1/2
  Radius/1 -> Mod/1  "driven  distance"

== system mount_2_rust/Mount_Drv_PDR2021/Parasitic torques model /Subsystem/Parasitic Torques/Parasitic EL ==
  MotTo : Inport
  MotPos : Inport  Port=2
  Cogging : Lookup_n-D  NumberOfTableDimensions=1  LookupTableObject=F_ripple  BreakpointsForDimension1=Pos  Table=Amp_Cog  InternalRulePriority=Speed  RndMeth=Simplest
  Constant : Constant  Value=0.1869
  Divide : Product  Inputs=**
  EMF Distortion : Lookup_n-D  NumberOfTableDimensions=1  LookupTableObject=F_ripple  BreakpointsForDimension1=Pos  Table=Amp_EMF  InternalRulePriority=Speed  RndMeth=Simplest
  Gain : Gain  Gain=1/R
  Gain1 : Gain  Gain=1/250
  Gain2 : Gain  Gain=1/N_Segm
  Mod1 : Math  Operator=rem  SignedPower=on
  Mod2 : Math  Operator=rem  SignedPower=on
  Radius : Gain  Gain=R
  Scope : Scope  Commented=on  NumInputPorts=2
  Sum : Sum  Inputs=|++
  Sum1 : Sum  Inputs=|++
  To : Outport
  wires:
  Mod2/1 -> EMF Distortion/1, Cogging/1
  Constant/1 -> Mod1/2, Sum1/2, Mod2/2
  Radius/1 -> Mod1/1  "driven distance"
  Mod1/1 -> Sum1/1
  Sum1/1 -> Mod2/1
  Gain1/1 -> Gain2/1  "I_rms"
  Gain2/1 -> Divide/1  "I_rms pro Segment"
  Divide/1 -> Sum/1, Scope/1
  EMF Distortion/1 -> Divide/2
  Gain/1 -> Gain1/1  "Force"
  MotTo/1 -> Gain/1
  Cogging/1 -> Sum/2, Scope/2
  Sum/1 -> To/1
  MotPos/1 -> Radius/1

== system mount_2_rust/Mount_Drv_PDR2021/Parasitic torques model /Subsystem/Parasitic Torques/Parasitic GIR ==
  MotTo : Inport
  MotPos : Inport  Port=2
  Cogging : Subsystem
  Emf : Subsystem
  Pretention : Constant  Value=T_pretension
  Product2 : Product  RndMeth=Zero
  Scope : Scope  Commented=on  NumInputPorts=2
  Sign : Signum  ZeroCross=off
  Sum1 : Sum  Inputs=|++
  Sum2 : Sum  Inputs=++|
  To : Outport
  wires:
  MotTo/1 -> Sum1/1, Sign/1
  Product2/1 -> Sum1/2
  Pretention/1 -> Product2/2
  Sign/1 -> Product2/1
  Sum1/1 -> Emf/1(To)
  Emf/1(T_emf) -> Sum2/1
  Cogging/1(T_cog) -> Sum2/2
  MotPos/1 -> Emf/2(Po), Cogging/1(Po)
  Sum2/1 -> To/1

== system mount_2_rust/Mount_Drv_PDR2021_Frless/Parasitic torques model /Subsystem/Parasitic Torques/Parasitic AZ ==
  MotTo : Inport
  MotPos : Inport  Port=2
  Cogging : Lookup_n-D  NumberOfTableDimensions=1  LookupTableObject=F_ripple  BreakpointsForDimension1=Pos  Table=Amp_Cog  InternalRulePriority=Speed  RndMeth=Simplest
  Constant : Constant  Value=0.1869
  Divide : Product  Inputs=**
  EMF Distortion : Lookup_n-D  NumberOfTableDimensions=1  LookupTableObject=F_ripple  BreakpointsForDimension1=Pos  Table=Amp_EMF  InternalRulePriority=Speed  RndMeth=Simplest
  Gain : Gain  Gain=1/R
  Gain1 : Gain  Gain=1/250
  Gain2 : Gain  Gain=1/N_Segm
  Mod : Math  Operator=rem  SignedPower=on
  Mod1 : Math  Operator=rem  SignedPower=on
  Radius : Gain  Gain=R
  Sum : Sum  Inputs=|++
  Sum1 : Sum  Inputs=|++
  To : Outport
  wires:
  Mod1/1 -> Cogging/1, EMF Distortion/1
  Sum1/1 -> Mod1/1
  Mod/1 -> Sum1/1
  Gain1/1 -> Gain2/1  "I_rms"
  Gain2/1 -> Divide/1  "I_rms pro Segment"
  Divide/1 -> Sum/1
  EMF Distortion/1 -> Divide/2
  Gain/1 -> Gain1/1  "Force"
  MotTo/1 -> Gain/1
  Cogging/1 -> Sum/2
  Sum/1 -> To/1
  MotPos/1 -> Radius/1
  Constant/1 -> Mod/2, Sum1/2, Mod1/2
  Radius/1 -> Mod/1  "driven  distance"

== system mount_2_rust/Mount_Drv_PDR2021_Frless/Parasitic torques model /Subsystem/Parasitic Torques/Parasitic EL ==
  MotTo : Inport
  MotPos : Inport  Port=2
  Cogging : Lookup_n-D  NumberOfTableDimensions=1  LookupTableObject=F_ripple  BreakpointsForDimension1=Pos  Table=Amp_Cog  InternalRulePriority=Speed  RndMeth=Simplest
  Constant : Constant  Value=0.1869
  Divide : Product  Inputs=**
  EMF Distortion : Lookup_n-D  NumberOfTableDimensions=1  LookupTableObject=F_ripple  BreakpointsForDimension1=Pos  Table=Amp_EMF  InternalRulePriority=Speed  RndMeth=Simplest
  Gain : Gain  Gain=1/R
  Gain1 : Gain  Gain=1/250
  Gain2 : Gain  Gain=1/N_Segm
  Mod1 : Math  Operator=rem  SignedPower=on
  Mod2 : Math  Operator=rem  SignedPower=on
  Radius : Gain  Gain=R
  Scope : Scope  Commented=on  NumInputPorts=2
  Sum : Sum  Inputs=|++
  Sum1 : Sum  Inputs=|++
  To : Outport
  wires:
  Mod2/1 -> EMF Distortion/1, Cogging/1
  Constant/1 -> Mod1/2, Sum1/2, Mod2/2
  Radius/1 -> Mod1/1  "driven distance"
  Mod1/1 -> Sum1/1
  Sum1/1 -> Mod2/1
  Gain1/1 -> Gain2/1  "I_rms"
  Gain2/1 -> Divide/1  "I_rms pro Segment"
  Divide/1 -> Sum/1, Scope/1
  EMF Distortion/1 -> Divide/2
  Gain/1 -> Gain1/1  "Force"
  MotTo/1 -> Gain/1
  Cogging/1 -> Sum/2, Scope/2
  Sum/1 -> To/1
  MotPos/1 -> Radius/1

== system mount_2_rust/Mount_Drv_PDR2021_Frless/Parasitic torques model /Subsystem/Parasitic Torques/Parasitic GIR ==
  MotTo : Inport
  MotPos : Inport  Port=2
  Cogging : Subsystem
  Emf : Subsystem
  Pretention : Constant  Value=T_pretension
  Product2 : Product  RndMeth=Zero
  Scope : Scope  Commented=on  NumInputPorts=2
  Sign : Signum  ZeroCross=off
  Sum1 : Sum  Inputs=|++
  Sum2 : Sum  Inputs=++|
  To : Outport
  wires:
  MotTo/1 -> Sum1/1, Sign/1
  Product2/1 -> Sum1/2
  Pretention/1 -> Product2/2
  Sign/1 -> Product2/1
  Sum1/1 -> Emf/1(To)
  Emf/1(T_emf) -> Sum2/1
  Cogging/1(T_cog) -> Sum2/2
  MotPos/1 -> Emf/2(Po), Cogging/1(Po)
  Sum2/1 -> To/1

== system mount_2_rust/Mount_Drv_PDR2021/ODC CT LUGRE Fr model/Friction/Friction Alt/g(v)/gs ==
  v : Inport
  Enable : EnablePort
  Divide : Product  Inputs=**
  Gain : Gain  Gain=1/vs
  Math Function : Math  SignedPower=on
  Math Function1 : Math  Operator=magnitude^2  SignedPower=on
  Unary Minus : UnaryMinus
  gs : Constant  Value=(Ts-Tc)/sigma0
  gs(v) : Outport
  wires:
  Divide/1 -> gs(v)/1
  v/1 -> Gain/1
  Gain/1 -> Math Function1/1
  Unary Minus/1 -> Math Function/1
  Math Function1/1 -> Unary Minus/1
  gs/1 -> Divide/2
  Math Function/1 -> Divide/1

== system mount_2_rust/Mount_Drv_PDR2021/ODC CT LUGRE Fr model/Friction/Friction Az/g(v)/gs ==
  v : Inport
  Enable : EnablePort
  Divide : Product  Inputs=**
  Gain : Gain  Gain=1/vs
  Math Function : Math  SignedPower=on
  Math Function1 : Math  Operator=magnitude^2  SignedPower=on
  Unary Minus : UnaryMinus
  gs : Constant  Value=(Ts-Tc)/sigma0
  gs(v) : Outport
  wires:
  Divide/1 -> gs(v)/1
  v/1 -> Gain/1
  Gain/1 -> Math Function1/1
  Unary Minus/1 -> Math Function/1
  Math Function1/1 -> Unary Minus/1
  gs/1 -> Divide/2
  Math Function/1 -> Divide/1

== system mount_2_rust/Mount_Drv_PDR2021/ODC CT LUGRE Fr model/Friction/Friction Gir/g(v)/gs ==
  v : Inport
  Enable : EnablePort
  Divide : Product  Inputs=**
  Gain : Gain  Gain=1/vs
  Math Function : Math  SignedPower=on
  Math Function1 : Math  Operator=magnitude^2  SignedPower=on
  Unary Minus : UnaryMinus
  gs : Constant  Value=(Ts-Tc)/sigma0
  gs(v) : Outport
  wires:
  Divide/1 -> gs(v)/1
  v/1 -> Gain/1
  Gain/1 -> Math Function1/1
  Unary Minus/1 -> Math Function/1
  Math Function1/1 -> Unary Minus/1
  gs/1 -> Divide/2
  Math Function/1 -> Divide/1

== system mount_2_rust/Mount_Drv_PDR2021/Parasitic torques model /Subsystem/Parasitic Torques/Parasitic GIR/Cogging ==
  Po : Inport
  CogAmp : Constant  Value=cog_amp
  CogSpatFreq : Constant  Value=cog_sfr
  Product1 : Product  RndMeth=Zero
  Product2 : Product  RndMeth=Zero
  Trigonometric Function : Trigonometry
  T_cog : Outport
  wires:
  Product2/1 -> T_cog/1
  Po/1 -> Product1/1
  Trigonometric Function/1 -> Product2/1
  CogAmp/1 -> Product2/2
  CogSpatFreq/1 -> Product1/2
  Product1/1 -> Trigonometric Function/1

== system mount_2_rust/Mount_Drv_PDR2021/Parasitic torques model /Subsystem/Parasitic Torques/Parasitic GIR/Emf ==
  To : Inport
  Po : Inport  Port=2
  EmfAmpFactor : Constant  Value=emf_ampFact
  EmfSpatFreq : Constant  Value=emf_sfr
  Product1 : Product  RndMeth=Zero
  Product2 : Product  Inputs=3  RndMeth=Zero
  Trigonometric Function : Trigonometry
  T_emf : Outport
  wires:
  To/1 -> Product2/3
  Product2/1 -> T_emf/1
  Po/1 -> Product1/1
  Trigonometric Function/1 -> Product2/1
  EmfAmpFactor/1 -> Product2/2
  EmfSpatFreq/1 -> Product1/2
  Product1/1 -> Trigonometric Function/1

== system mount_2_rust/Mount_Drv_PDR2021_Frless/Parasitic torques model /Subsystem/Parasitic Torques/Parasitic GIR/Cogging ==
  Po : Inport
  CogAmp : Constant  Value=cog_amp
  CogSpatFreq : Constant  Value=cog_sfr
  Product1 : Product  RndMeth=Zero
  Product2 : Product  RndMeth=Zero
  Trigonometric Function : Trigonometry
  T_cog : Outport
  wires:
  Product2/1 -> T_cog/1
  Po/1 -> Product1/1
  Trigonometric Function/1 -> Product2/1
  CogAmp/1 -> Product2/2
  CogSpatFreq/1 -> Product1/2
  Product1/1 -> Trigonometric Function/1

== system mount_2_rust/Mount_Drv_PDR2021_Frless/Parasitic torques model /Subsystem/Parasitic Torques/Parasitic GIR/Emf ==
  To : Inport
  Po : Inport  Port=2
  EmfAmpFactor : Constant  Value=emf_ampFact
  EmfSpatFreq : Constant  Value=emf_sfr
  Product1 : Product  RndMeth=Zero
  Product2 : Product  Inputs=3  RndMeth=Zero
  Trigonometric Function : Trigonometry
  T_emf : Outport
  wires:
  To/1 -> Product2/3
  Product2/1 -> T_emf/1
  Po/1 -> Product1/1
  Trigonometric Function/1 -> Product2/1
  EmfAmpFactor/1 -> Product2/2
  EmfSpatFreq/1 -> Product1/2
  Product1/1 -> Trigonometric Function/1
